simulink model "chap8_2sim"  (Simulink 8.1)
settings: Solver=ode45  StartTime=0.0  StopTime=150  RelTol=1e-3
settings Model: Creator=liujk  LastModifiedBy=liujk  ExtModeTrigMode=oneshot  ExtModeArmWhenConnect=off
settings DataIOCC: LimitDataPoints=off  SignalLoggingName=sigsOut
settings OptimizationCC: BooleanDataType=off  ExpressionDepthLimit=128
settings DebuggingCC: SaveWithParameterizedLinksMsg=none  SignalResolutionControl=TryResolveAllWithWarning  SolverPrmCheckMsg=none  MultiTaskDSMMsg=warning  MultiTaskCondExecSysMsg=none  FcnCallInpInsideContextMsg=EnableAllAsError  StrictBusMsg=None
settings HardwareCC: TargetUnknown=on
settings RTWCC: IncludeERTFirstTime=on

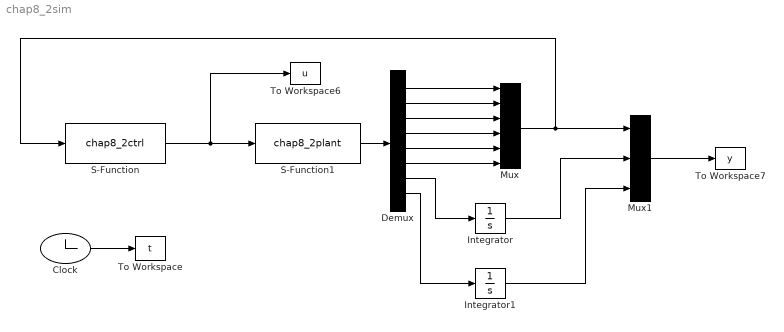
== system chap8_2sim ==
  Clock : Clock
  Demux : Demux  Outputs=8
  Integrator : Integrator
  Integrator1 : Integrator
  Mux : Mux  Inputs=6
  Mux1 : Mux  Inputs=3
  S-Function : S-Function  FunctionName=chap8_2ctrl  EnableBusSupport=off
  S-Function1 : S-Function  FunctionName=chap8_2plant  EnableBusSupport=off
  To Workspace : ToWorkspace  VariableName=t  SampleTime=-1
  To Workspace6 : ToWorkspace  VariableName=u  SampleTime=-1
  To Workspace7 : ToWorkspace  VariableName=y  SampleTime=-1
  wires:
  S-Function/1 -> S-Function1/1, To Workspace6/1
  Clock/1 -> To Workspace/1
  S-Function1/1 -> Demux/1
  Demux/1 -> Mux/1
  Demux/2 -> Mux/2
  Demux/3 -> Mux/3
  Demux/4 -> Mux/4
  Demux/5 -> Mux/5
  Demux/6 -> Mux/6
  Demux/7 -> Integrator/1
  Demux/8 -> Integrator1/1
  Mux/1 -> Mux1/1, S-Function/1
  Integrator/1 -> Mux1/2
  Integrator1/1 -> Mux1/3
  Mux1/1 -> To Workspace7/1
